simulink model "sub_test"  (R2017a)
settings: Solver=FixedStepDiscrete  StartTime=0.0  StopTime=10.0  RelTol=1e-3
settings Model: Creator=rober  LastModifiedBy=rober
settings ConfigComp: PLC_TargetIDE=plcopen  PLC_GenerateReport=off

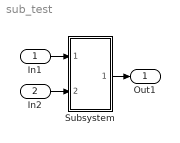
== system sub_test ==
  In1 : Inport
  In2 : Inport  Port=2
  Subsystem : Subsystem  TreatAsAtomicUnit=on
  Out1 : Outport
  wires:
  In1/1 -> Subsystem/1(In1)
  In2/1 -> Subsystem/2(In2)
  Subsystem/1(Out1) -> Out1/1

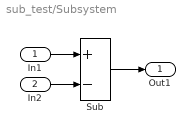
== system sub_test/Subsystem ==
  In1 : Inport
  In2 : Inport  Port=2
  Sub : Sum  Inputs=+-
  Out1 : Outport
  wires:
  Sub/1 -> Out1/1
  In1/1 -> Sub/1
  In2/1 -> Sub/2
